simulink model "graduation_project_prototype_collect_4"  (R2023a)
settings: Solver=VariableStepAuto  StartTime=0.0  StopTime=2  MaxStep=5e-3  RelTol=1e-3
libraries: spsFourierLib x10, slpidlib x3, spsAsynchronousMachineSIUnitsLib x1, spsDCVoltageSourceLib x1, spsPWMGenerator2LevelLib x1, spsSVPWMGenerator2LevelLib x1, spsabctoAlphaBetaZeroLib x1, spsabctodq0Lib x1, spsdq0toAlphaBetaZeroLib x1, spsThreePhaseVIMeasurementLib x1, spsTwoLevelConverterLib x1, sps_lib x1
settings Model: SimulationMode=accelerator  Creator=ehabt  LastModifiedBy=mohammed
settings DataIOCC: SaveOutput=off  SignalLogging=off  DSMLogging=off  SaveTime=off  ReturnWorkspaceOutputs=off

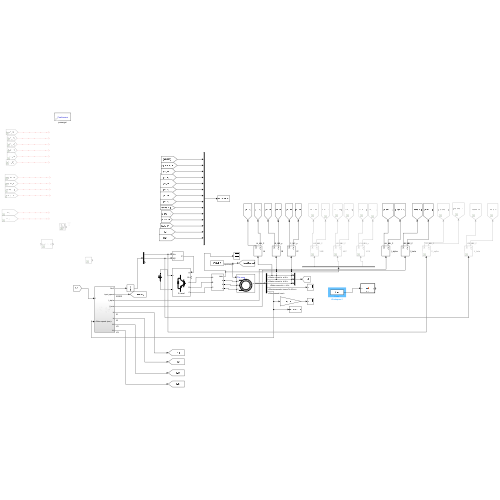
[thumbnail: Simulink's stored preview of the top-level diagram]
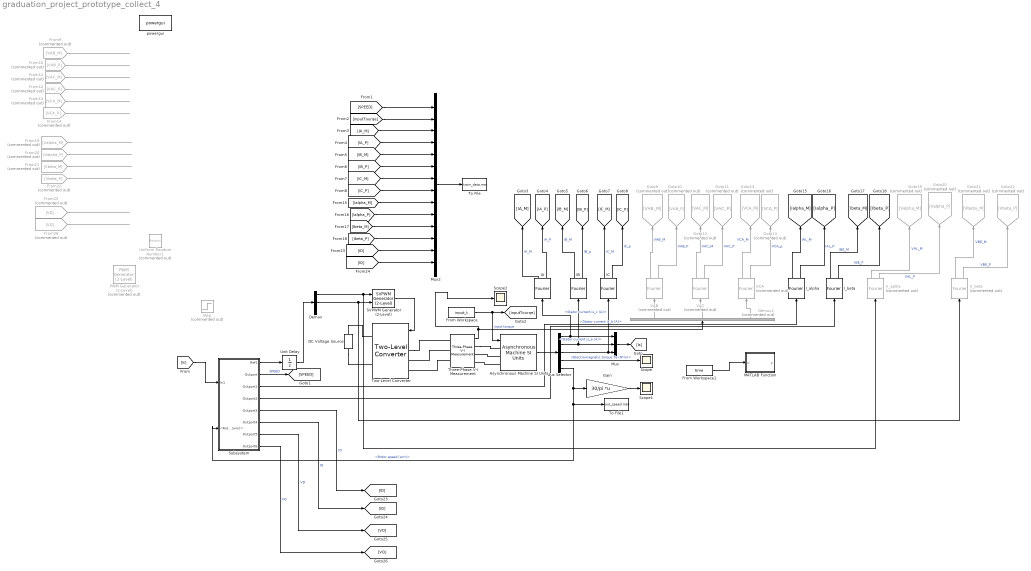
== system graduation_project_prototype_collect_4 ==
  Asynchronous Machine SI Units : spsAsynchronousMachineSIUnitsLib/Asynchronous Machine SI Units  RotorType=Squirrel-cage  PresetModel=No  MechanicalLoad=Torque Tm  ShowDetailedParameters=on  ReferenceFrame=Rotor  Units=SI  MeasurementBus=off  NominalParameters=[4000 400 50]  VoltageRatio=1  Stator=[1.405 0.005839]  Rotor=[1.395 0.005839]  Cage1=[0.4155 0.002066]  Cage2=[0.4168 0.0003495]  Lm=0.1722  Mechanical=[0.0131*3 0.002985 2]  PolePairs=2  InitialConditions=[1 0 0 0 0 0 0 0]  SimulateSaturation=off  Saturation=[14.03593122, 27.81365428, 53.79336849, 72.68890987, 97.98006896, 148.6815601, 215.7428561, 302.9841135, 428.7778367 ; 230, 322, 414, 460, 506, 552, 598, 644, 690]  LoadFlowParameters=1492000  TsPowergui=0  TsBlock=-1  IterativeModel=Trapezoidal non iterative  IterativeDiscreteModel=Trapezoidal non iterative  Pmec=1.492e+006
  Bus Selector : BusSelector  OutputSignals=Stator measurements.Stator current is_a (A),Stator measurements.Stator current is_b (A),Stator measurements.Stator current is_c (A),Mechanical.Electromagnetic torque Te (N*m),Mechanical.Rotor speed (wm)
  DC Voltage Source : spsDCVoltageSourceLib/DC Voltage Source  Amplitude=660  Measurements=None
  Demux : Demux  Outputs=3
  Demux1 : Demux  Commented=on  Outputs=3
  From Workspace : FromWorkspace  VariableName=input_t  SampleTime=2
  From Workspace1 : FromWorkspace  VariableName=time  SampleTime=1
  From10 : From  Commented=on  GotoTag=VAB_P
  From11 : From  Commented=on  GotoTag=VAC_M
  From12 : From  Commented=on  GotoTag=VAC_P
  From13 : From  Commented=on  GotoTag=VCA_M
  From14 : From  Commented=on  GotoTag=VCA_P
  From19 : From  Commented=on  GotoTag=Valpha_M
  From20 : From  Commented=on  GotoTag=Valpha_P
  From21 : From  Commented=on  GotoTag=Vbeta_M
  From22 : From  Commented=on  GotoTag=Vbeta_P
  From25 : From  Commented=on  GotoTag=VD
  From26 : From  Commented=on  GotoTag=VQ
  From9 : From  Commented=on  GotoTag=VAB_M
  Gain : Gain  Gain=30/pi  Multiplication=Matrix(K*u)
  Goto10 : Goto  Commented=on  GotoTag=VAB_P
  Goto11 : Goto  Commented=on  GotoTag=VAC_P
  Goto12 : Goto  Commented=on  GotoTag=VAC_M
  Goto13 : Goto  Commented=on  GotoTag=VCA_P
  Goto14 : Goto  Commented=on  GotoTag=VCA_M
  Goto19 : Goto  Commented=on  GotoTag=Valpha_M
  Goto20 : Goto  Commented=on  GotoTag=Valpha_P
  Goto21 : Goto  Commented=on  GotoTag=Vbeta_M
  Goto22 : Goto  Commented=on  GotoTag=Vbeta_P
  Goto9 : Goto  Commented=on  GotoTag=VAB_M
  IA : spsFourierLib/Fourier  Freq=50  n=1  InInit=[0, 0]  Ts=0
  IB : spsFourierLib/Fourier  Freq=50  n=1  InInit=[0, 0]  Ts=0
  IC : spsFourierLib/Fourier  Freq=50  n=1  InInit=[0, 0]  Ts=0
  I_alpha : spsFourierLib/Fourier  Freq=50  n=1  InInit=[0, 0]  Ts=0
  I_beta : spsFourierLib/Fourier  Freq=50  n=1  InInit=[0, 0]  Ts=0
  MATLAB Function : MATLAB Function  TreatAsAtomicUnit=on
  Mux : Mux  Inputs=3
  Mux2 : Mux  Inputs=14
  PWM Generator (2-Level) : spsPWMGenerator2LevelLib/PWM Generator (2-Level)  Commented=on  ModulatorType=Three-phase bridge (6 pulses)  ModulatorMode=Unsynchronized  Fc=5000  Pc=90  nF=27  MinMax="[ -1  1 ]"  SamplingTechnique=Natural  ModulatingSignals=off  m=0.8  Freq=60  Phase=0  Ts=0  ShowCarrierOutport=off
  SVPWM Generator (2-Level) : spsSVPWMGenerator2LevelLib/SVPWM Generator (2-Level)  InputType=alpha-beta components  SwitchingPattern=Pattern #1  Fc=15000  ParUref=[0.8 -30 50]  Ts=0
  Scope : Scope
  Scope1 : Scope
  Scope2 : Scope
  Step : Step  Commented=on  After=26  SampleTime=0
  Subsystem : Subsystem
  Three-Phase V-I Measurement : spsThreePhaseVIMeasurementLib/Three-Phase V-I Measurement  VoltageMeasurement=phase-to-phase  SetLabelV=off  LabelV=Vabc  Vpu=off  VpuLL=off  CurrentMeasurement=no  SetLabelI=off  LabelI=Iabc  Ipu=off  Pbase=100e6  Vbase=500e3  OutputType=Complex  PhasorSimulation=off  PSBequivalent=0
  To File : ToFile  Filename=train_data.mat  MatrixName=train_data  SaveFormat=Timeseries  SampleTime=1.99
  To File1 : ToFile  Filename=out_speed.mat  MatrixName=out_speed  SaveFormat=Timeseries  SampleTime=1.99
  Two-Level Converter : spsTwoLevelConverterLib/Two-Level Converter  ModelType=Switching devices  Ron=1e-3  Rs=1e6  Cs=inf  Vforward=[0,0]  Ron_Diode=1e-3  Rs_Diode=1e6  Cs_Diode=inf  Vf_Diode=1e-3  Rs_CurrentSource=inf  Ron_ACsource=1e-3
      settings: LibrarySourceBlock=sps_lib/Power Electronics/Two-Level Converter
  Uniform Random Number1 : UniformRandomNumber  Commented=on  Minimum=0  Maximum=26  Seed=1234  SampleTime=2
  Unit Delay : UnitDelay  SampleTime=-1  HasFrameUpgradeWarning=on
  VAB : spsFourierLib/Fourier  Commented=on  Freq=50  n=1  InInit=[0, 0]  Ts=0
  VAC : spsFourierLib/Fourier  Commented=on  Freq=50  n=1  InInit=[0, 0]  Ts=0
  VCA : spsFourierLib/Fourier  Commented=on  Freq=50  n=1  InInit=[0, 0]  Ts=0
  V_aplha : spsFourierLib/Fourier  Commented=on  Freq=50  n=1  InInit=[0, 0]  Ts=0
  V_beta : spsFourierLib/Fourier  Commented=on  Freq=50  n=1  InInit=[0, 0]  Ts=0
  powergui : sps_lib/powergui  Priority=1  SimulationMode=Continuous  SampleTime=50e-6  frequency=60  Iterations=50  frequencyindice=50  Pbase=100e6  ErrMax=1e-4  UnitsV=kV  UnitsW=MW  buscounter=0  FunctionMessages=off  echomessages=off  EnableUseOfTLC=off  CurrentSourceSwitches=off  DisableSnubberDevices=off  DisableRonSwitches=off  DisableVfSwitches=off  DisplayEquations=off  AutomaticDiscreteSolvers=off  SolverType=Tustin/Backward Euler (TBE)  Interpol=off  ExternalGateDelay=off  methode=off  Ts=100  x0status=blocks  SPID=on  SwTol=0  HookPort=off  NonlinearTolerance=1e-4  nMaxIteration=100  ContinueOnMaxIteration=off  RestoreLinks=warning  ResistiveCurrentMeasurement=off  Frange=[0:2:500]  Ylog=off  Xlog=on  ShowGrid=off  save=off  variable=ZData  structure=0  ZoomFFT=off  StartTime=0.0  cycles=1  DisplayStyle=1  fundamental=60  FreqAxis=off  MaxFrequency=1000  frequencyindicesteady=1  RmsSteady=1  display=off
  wires:
  Asynchronous Machine SI Units/1 -> Bus Selector/1
  Bus Selector/1 -> Mux/1, IA/1  "<Stator current is_a (A)>"
  Bus Selector/2 -> Mux/2, IB/1  "<Stator current is_b (A)>"
  Bus Selector/3 -> IC/1, Mux/3  "<Stator current is_c (A)>"
  Bus Selector/4 -> Scope/1  "<Electromagnetic torque Te (N*m)>"
  Mux/1 -> [Is]
  Bus Selector/5 -> To File1/1, Subsystem/2(<Rotor speed (wm)>), Gain/1  "<Rotor speed (wm)>"
  Gain/1 -> Scope1/1
  [Is] -> Subsystem/1(In1)
  Three-Phase V-I Measurement/1 -> Demux1/1, Scope2/1
  Subsystem/1(Ref1) -> Unit Delay/1
  Unit Delay/1 -> Demux/1
  Demux/1 -> V_aplha/1, SVPWM Generator (2-Level)/1
  Demux/2 -> V_beta/1, SVPWM Generator (2-Level)/2
  SVPWM Generator (2-Level)/1 -> Two-Level Converter/1
  From Workspace/1 -> Asynchronous Machine SI Units/1, [inputTourqe]  "input torque"
  Demux1/1 -> VAB/1
  Demux1/2 -> VAC/1
  Demux1/3 -> VCA/1
  Subsystem/3(Outport1) -> I_alpha/1
  Subsystem/4(Outport2) -> I_beta/1
  Subsystem/2(Outport) -> [SPEED]  "SPEED"
  [SPEED] -> Mux2/1
  [inputTourqe] -> Mux2/2
  IA/1 -> [IA_M]  "IA_M"
  IA/2 -> [IA_P]  "IA_P"
  IB/1 -> [IB_M]  "IB_M"
  IB/2 -> [IB_P]  "IB_p"
  IC/1 -> [IC_M]  "IC_M"
  IC/2 -> [IC_P]  "IC_p"
  VAB/1 -> Goto9/1  "VAB_M"
  VAB/2 -> Goto10/1  "VAB_P"
  VAC/1 -> Goto12/1  "VAC_M"
  VAC/2 -> Goto11/1  "VAC_P"
  VCA/1 -> Goto14/1  "VCA_M"
  VCA/2 -> Goto13/1  "VCA_p"
  I_alpha/1 -> [Ialpha_M]  "IAL_M"
  I_alpha/2 -> [Ialpha_P]  "IAL_P"
  I_beta/1 -> [Ibeta_M]  "IBE_M"
  I_beta/2 -> [Ibeta_P]  "IBE_P"
  V_aplha/1 -> Goto19/1  "VAL_M"
  V_aplha/2 -> Goto20/1  "VAL_P"
  V_beta/1 -> Goto21/1  "VBE_M"
  V_beta/2 -> Goto22/1  "VBE_P"
  Subsystem/5(Outport3) -> [ID]  "ID"
  Subsystem/6(Outport4) -> [IQ]  "IQ"
  Subsystem/7(Outport5) -> [VD]  "VD"
  Subsystem/8(Outport6) -> [VQ]  "VQ"
  [IA_M] -> Mux2/3
  [IA_P] -> Mux2/4
  [IB_M] -> Mux2/5
  [IB_P] -> Mux2/6
  [IC_M] -> Mux2/7
  [IC_P] -> Mux2/8
  From9/1 -> ?
  From10/1 -> ?
  From11/1 -> ?
  From12/1 -> ?
  From13/1 -> ?
  From14/1 -> ?
  [Ialpha_M] -> Mux2/9
  [Ialpha_P] -> Mux2/10
  [Ibeta_M] -> Mux2/11
  [Ibeta_P] -> Mux2/12
  From19/1 -> ?
  From20/1 -> ?
  From21/1 -> ?
  From22/1 -> ?
  [ID] -> Mux2/13
  [IQ] -> Mux2/14
  From25/1 -> ?
  From26/1 -> ?
  Mux2/1 -> To File/1
  From Workspace1/1 -> MATLAB Function/1(u)
  connections:
  Asynchronous Machine SI Units/LConn2 -- Three-Phase V-I Measurement/RConn2
  Asynchronous Machine SI Units/LConn3 -- Three-Phase V-I Measurement/RConn3
  DC Voltage Source/RConn1 -- Two-Level Converter/RConn1
  DC Voltage Source/LConn1 -- Two-Level Converter/RConn2
  Three-Phase V-I Measurement/LConn2 -- Two-Level Converter/LConn2
  Three-Phase V-I Measurement/LConn3 -- Two-Level Converter/LConn3
  Three-Phase V-I Measurement/RConn1 -- Asynchronous Machine SI Units/LConn1
  Two-Level Converter/LConn1 -- Three-Phase V-I Measurement/LConn1

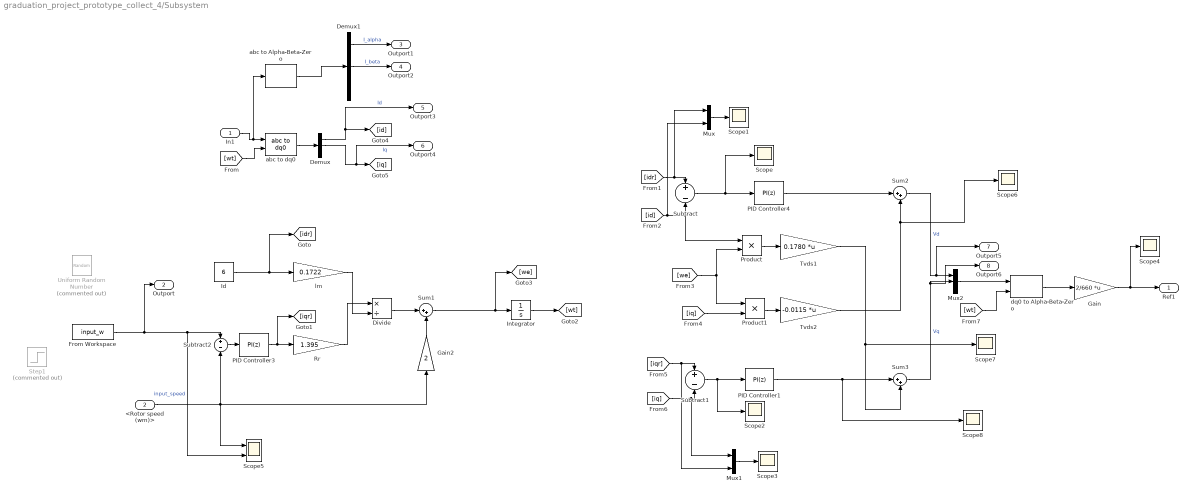
== system graduation_project_prototype_collect_4/Subsystem ==
  In1 : Inport
  <Rotor speed (wm)> : Inport  Port=2
  Demux : Demux  Outputs=3
  Demux1 : Demux  Outputs=3
  Divide : Product  Inputs=*/
  From Workspace : FromWorkspace  VariableName=input_w  SampleTime=2
  Gain : Gain  Gain=2/660  Multiplication=Matrix(K*u)
  Gain2 : Gain  Gain=2
  Id : Constant  Value=6
  Integrator : Integrator
  Mux : Mux  Inputs=2
  Mux1 : Mux  Inputs=2
  Mux2 : Mux  Inputs=3
  PID Controller1 : slpidlib/PID Controller  Controller=PI  Form=Parallel  TimeDomain=Discrete-time  UseExternalTs=off  SampleTime=100e-6  IntegratorMethod=Forward Euler  FilterMethod=Forward Euler  ControllerParametersSource=internal  P=6.66265142907135  I=1139.27458602713  UseKiTs=off  D=0  N=100  UseFilter=on  TunerSelectOption=Transfer Function Based (PID Tuner App)  InitialConditionSource=internal  InitialConditionForIntegrator=0  InitialConditionForFilter=0  DifferentiatorICPrevScaledInput=0  ExternalReset=none  TrackingMode=off  Kt=1  LimitOutput=on  SatLimitsSource=internal  UpperSaturationLimit=330  LowerSaturationLimit=-330  LinearizeAsGain=on  AntiWindupMode=clamping  Kb=1  LimitIntegrator=off  UpperIntegratorSaturationLimit=inf  LowerIntegratorSaturationLimit=-inf  POutMin=[]  POutMax=[]  IOutMin=[]  IOutMax=[]  DOutMin=[]  DOutMax=[]  NOutMin=[]  NOutMax=[]  SumOutMin=[]  SumOutMax=[]  SaturationOutMin=[]  SaturationOutMax=[]  PParamMin=[]  PParamMax=[]  IParamMin=[]  IParamMax=[]  DParamMin=[]  DParamMax=[]  NParamMin=[]  NParamMax=[]  KbParamMin=[]  KbParamMax=[]  KtParamMin=[]  KtParamMax=[]  KbOutMin=[]  KbOutMax=[]  KtOutMin=[]  KtOutMax=[]  IntegratorOutMin=[]  IntegratorOutMax=[]  FilterOutMin=[]  FilterOutMax=[]  SumI1OutMin=[]  SumI1OutMax=[]  SumI2OutMin=[]  SumI2OutMax=[]  SumI3OutMin=[]  SumI3OutMax=[]  SumI4OutMin=[]  SumI4OutMax=[]  SumDOutMin=[]  SumDOutMax=[]  DifferentiatorOutMin=[]  DifferentiatorOutMax=[]  FilterDiffOutCoefMin=[]  FilterDiffOutCoefMax=[]  ReciprocalOutMin=[]  ReciprocalOutMax=[]  SumDenOutMin=[]  SumDenOutMax=[]  SumNumOutMin=[]  SumNumOutMax=[]  DivideOutMin=[]  DivideOutMax=[]  UdiffTsProdOutMin=[]  UdiffTsProdOutMax=[]  NTsProdOutMin=[]  NTsProdOutMax=[]  UintegralTsProdOutMin=[]  UintegralTsProdOutMax=[]  UngainTsProdOutMin=[]  UngainTsProdOutMax=[]  ClampingZeroOutDataTypeStr=Inherit: Inherit via back propagation  ClampingZeroOutMin=[]  ClampingZeroOutMax=[]  FilterDenConstantOutDataTypeStr=Inherit: Inherit via back propagation  FilterDenConstantOutMin=[]  FilterDenConstantOutMax=[]  PCopyOutDataTypeStr=Inherit: Inherit via back propagation  PCopyOutMin=[]  PCopyOutMax=[]  NCopyOutDataTypeStr=Inherit: Inherit via back propagation  NCopyOutMin=[]  NCopyOutMax=[]  IntegratorContinuousStateAttributes=''  IntegratorStateMustResolveToSignalObject=off  IntegratorRTWStateStorageClass=Auto  FilterContinuousStateAttributes=''  FilterStateMustResolveToSignalObject=off  FilterRTWStateStorageClass=Auto  ParallelPVariant=InternalParameters  IdealPVariant=Disabled  IVariant=InternalParameters  DVariant=Disabled  IntegratorVariant=Discrete  SatVariant=Enabled  AWVariant=DiscClampingParallel  PCopyVariant=Disabled  TRVariant=Disabled  FdbkBlocksVariant=Forward  IdealPFdbkVariant=Disabled  SatFdbkVariant=Disabled  DerivativeFilterVariant=Disabled  NVariant=Disabled  NCopyVariant=Disabled_SignalSpec  FilterICVariant=Disabled  IntegratorICVariant=InternalICs  ExternalResetVariant=Disabled  TRSumVariant=Passthrough  SumFdbkVariant=Disabled  SumVariant=Sum_PI  TsampFilterVariant=InternalTs  TsampNgainVariant=Passthrough  TsampIntegralVariant=Disabled_SignalSpec  ExternalSaturationOutDataTypeStr=Inherit: Same as second input
  PID Controller3 : slpidlib/PID Controller  Controller=PI  Form=Parallel  TimeDomain=Discrete-time  UseExternalTs=off  SampleTime=100e-6  IntegratorMethod=Forward Euler  FilterMethod=Forward Euler  ControllerParametersSource=internal  P=1.27476437850265  I=15.6272018921627  UseKiTs=off  D=0  N=100  UseFilter=on  TunerSelectOption=Transfer Function Based (PID Tuner App)  InitialConditionSource=internal  InitialConditionForIntegrator=0  InitialConditionForFilter=0  DifferentiatorICPrevScaledInput=0  ExternalReset=none  TrackingMode=off  Kt=1  LimitOutput=on  SatLimitsSource=internal  UpperSaturationLimit=18  LowerSaturationLimit=-18  LinearizeAsGain=on  AntiWindupMode=clamping  Kb=1  LimitIntegrator=off  UpperIntegratorSaturationLimit=inf  LowerIntegratorSaturationLimit=-inf  POutMin=[]  POutMax=[]  IOutMin=[]  IOutMax=[]  DOutMin=[]  DOutMax=[]  NOutMin=[]  NOutMax=[]  SumOutMin=[]  SumOutMax=[]  SaturationOutMin=[]  SaturationOutMax=[]  PParamMin=[]  PParamMax=[]  IParamMin=[]  IParamMax=[]  DParamMin=[]  DParamMax=[]  NParamMin=[]  NParamMax=[]  KbParamMin=[]  KbParamMax=[]  KtParamMin=[]  KtParamMax=[]  KbOutMin=[]  KbOutMax=[]  KtOutMin=[]  KtOutMax=[]  IntegratorOutMin=[]  IntegratorOutMax=[]  FilterOutMin=[]  FilterOutMax=[]  SumI1OutMin=[]  SumI1OutMax=[]  SumI2OutMin=[]  SumI2OutMax=[]  SumI3OutMin=[]  SumI3OutMax=[]  SumI4OutMin=[]  SumI4OutMax=[]  SumDOutMin=[]  SumDOutMax=[]  DifferentiatorOutMin=[]  DifferentiatorOutMax=[]  FilterDiffOutCoefMin=[]  FilterDiffOutCoefMax=[]  ReciprocalOutMin=[]  ReciprocalOutMax=[]  SumDenOutMin=[]  SumDenOutMax=[]  SumNumOutMin=[]  SumNumOutMax=[]  DivideOutMin=[]  DivideOutMax=[]  UdiffTsProdOutMin=[]  UdiffTsProdOutMax=[]  NTsProdOutMin=[]  NTsProdOutMax=[]  UintegralTsProdOutMin=[]  UintegralTsProdOutMax=[]  UngainTsProdOutMin=[]  UngainTsProdOutMax=[]  ClampingZeroOutDataTypeStr=Inherit: Inherit via back propagation  ClampingZeroOutMin=[]  ClampingZeroOutMax=[]  FilterDenConstantOutDataTypeStr=Inherit: Inherit via back propagation  FilterDenConstantOutMin=[]  FilterDenConstantOutMax=[]  PCopyOutDataTypeStr=Inherit: Inherit via back propagation  PCopyOutMin=[]  PCopyOutMax=[]  NCopyOutDataTypeStr=Inherit: Inherit via back propagation  NCopyOutMin=[]  NCopyOutMax=[]  IntegratorContinuousStateAttributes=''  IntegratorStateMustResolveToSignalObject=off  IntegratorRTWStateStorageClass=Auto  FilterContinuousStateAttributes=''  FilterStateMustResolveToSignalObject=off  FilterRTWStateStorageClass=Auto  ParallelPVariant=InternalParameters  IdealPVariant=Disabled  IVariant=InternalParameters  DVariant=Disabled  IntegratorVariant=Discrete  SatVariant=Enabled  AWVariant=DiscClampingParallel  PCopyVariant=Disabled  TRVariant=Disabled  FdbkBlocksVariant=Forward  IdealPFdbkVariant=Disabled  SatFdbkVariant=Disabled  DerivativeFilterVariant=Disabled  NVariant=Disabled  NCopyVariant=Disabled_SignalSpec  FilterICVariant=Disabled  IntegratorICVariant=InternalICs  ExternalResetVariant=Disabled  TRSumVariant=Passthrough  SumFdbkVariant=Disabled  SumVariant=Sum_PI  TsampFilterVariant=InternalTs  TsampNgainVariant=Passthrough  TsampIntegralVariant=Disabled_SignalSpec  ExternalSaturationOutDataTypeStr=Inherit: Same as second input
  PID Controller4 : slpidlib/PID Controller  Controller=PI  Form=Parallel  TimeDomain=Discrete-time  UseExternalTs=off  SampleTime=100e-6  IntegratorMethod=Forward Euler  FilterMethod=Forward Euler  ControllerParametersSource=internal  P=12.2885137139008  I=162.749993865987  UseKiTs=off  D=0  N=100  UseFilter=on  TunerSelectOption=Transfer Function Based (PID Tuner App)  InitialConditionSource=internal  InitialConditionForIntegrator=0  InitialConditionForFilter=0  DifferentiatorICPrevScaledInput=0  ExternalReset=none  TrackingMode=off  Kt=1  LimitOutput=on  SatLimitsSource=internal  UpperSaturationLimit=330  LowerSaturationLimit=-330  LinearizeAsGain=on  AntiWindupMode=clamping  Kb=1  LimitIntegrator=off  UpperIntegratorSaturationLimit=inf  LowerIntegratorSaturationLimit=-inf  POutMin=[]  POutMax=[]  IOutMin=[]  IOutMax=[]  DOutMin=[]  DOutMax=[]  NOutMin=[]  NOutMax=[]  SumOutMin=[]  SumOutMax=[]  SaturationOutMin=[]  SaturationOutMax=[]  PParamMin=[]  PParamMax=[]  IParamMin=[]  IParamMax=[]  DParamMin=[]  DParamMax=[]  NParamMin=[]  NParamMax=[]  KbParamMin=[]  KbParamMax=[]  KtParamMin=[]  KtParamMax=[]  KbOutMin=[]  KbOutMax=[]  KtOutMin=[]  KtOutMax=[]  IntegratorOutMin=[]  IntegratorOutMax=[]  FilterOutMin=[]  FilterOutMax=[]  SumI1OutMin=[]  SumI1OutMax=[]  SumI2OutMin=[]  SumI2OutMax=[]  SumI3OutMin=[]  SumI3OutMax=[]  SumI4OutMin=[]  SumI4OutMax=[]  SumDOutMin=[]  SumDOutMax=[]  DifferentiatorOutMin=[]  DifferentiatorOutMax=[]  FilterDiffOutCoefMin=[]  FilterDiffOutCoefMax=[]  ReciprocalOutMin=[]  ReciprocalOutMax=[]  SumDenOutMin=[]  SumDenOutMax=[]  SumNumOutMin=[]  SumNumOutMax=[]  DivideOutMin=[]  DivideOutMax=[]  UdiffTsProdOutMin=[]  UdiffTsProdOutMax=[]  NTsProdOutMin=[]  NTsProdOutMax=[]  UintegralTsProdOutMin=[]  UintegralTsProdOutMax=[]  UngainTsProdOutMin=[]  UngainTsProdOutMax=[]  ClampingZeroOutDataTypeStr=Inherit: Inherit via back propagation  ClampingZeroOutMin=[]  ClampingZeroOutMax=[]  FilterDenConstantOutDataTypeStr=Inherit: Inherit via back propagation  FilterDenConstantOutMin=[]  FilterDenConstantOutMax=[]  PCopyOutDataTypeStr=Inherit: Inherit via back propagation  PCopyOutMin=[]  PCopyOutMax=[]  NCopyOutDataTypeStr=Inherit: Inherit via back propagation  NCopyOutMin=[]  NCopyOutMax=[]  IntegratorContinuousStateAttributes=''  IntegratorStateMustResolveToSignalObject=off  IntegratorRTWStateStorageClass=Auto  FilterContinuousStateAttributes=''  FilterStateMustResolveToSignalObject=off  FilterRTWStateStorageClass=Auto  ParallelPVariant=InternalParameters  IdealPVariant=Disabled  IVariant=InternalParameters  DVariant=Disabled  IntegratorVariant=Discrete  SatVariant=Enabled  AWVariant=DiscClampingParallel  PCopyVariant=Disabled  TRVariant=Disabled  FdbkBlocksVariant=Forward  IdealPFdbkVariant=Disabled  SatFdbkVariant=Disabled  DerivativeFilterVariant=Disabled  NVariant=Disabled  NCopyVariant=Disabled_SignalSpec  FilterICVariant=Disabled  IntegratorICVariant=InternalICs  ExternalResetVariant=Disabled  TRSumVariant=Passthrough  SumFdbkVariant=Disabled  SumVariant=Sum_PI  TsampFilterVariant=InternalTs  TsampNgainVariant=Passthrough  TsampIntegralVariant=Disabled_SignalSpec  ExternalSaturationOutDataTypeStr=Inherit: Same as second input
  Product : Product
  Product1 : Product
  Rr : Gain  Gain=1.395
  Scope{,1..4,6..8} (8 alike) : Scope
  Scope5 : Scope  NumInputPorts=2
  Step1 : Step  Commented=on  Time=0.2  After=1250*pi/30  SampleTime=0
  Subtract : Sum  Inputs=+-
  Subtract1 : Sum  Inputs=+-
  Subtract2 : Sum  Inputs=+-
  Sum1 : Sum  Inputs=|++
  Sum2 : Sum  Inputs=|++
  Sum3 : Sum  Inputs=|++
  Tvds1 : Gain  Gain=0.1780  Multiplication=Matrix(K*u)
  Tvds2 : Gain  Gain=-0.0115  Multiplication=Matrix(K*u)
  Uniform Random Number : UniformRandomNumber  Commented=on  Minimum=0  Maximum=1500*pi/30  Seed=1234  SampleTime=2
  abc to Alpha-Beta-Zero : spsabctoAlphaBetaZeroLib/abc to Alpha-Beta-Zero
  abc to dq0 : spsabctodq0Lib/abc to dq0  Alignment=90 degrees behind phase A axis
  dq0 to Alpha-Beta-Zero : spsdq0toAlphaBetaZeroLib/dq0 to Alpha-Beta-Zero  Alignment=90 degrees behind phase A axis
  lm : Gain  Gain=0.1722
  Ref1 : Outport
  Outport : Outport  Port=2
  Outport1 : Outport  Port=3
  Outport2 : Outport  Port=4
  Outport3 : Outport  Port=5
  Outport4 : Outport  Port=6
  Outport5 : Outport  Port=7
  Outport6 : Outport  Port=8
  wires:
  <Rotor speed (wm)>/1 -> Subtract2/2, Scope5/1, Gain2/1
  Rr/1 -> Divide/1
  Id/1 -> [idr], lm/1
  lm/1 -> Divide/2
  Divide/1 -> Sum1/1
  Sum1/1 -> [we], Integrator/1
  Integrator/1 -> [wt]
  Subtract2/1 -> PID Controller3/1
  PID Controller3/1 -> [iqr], Rr/1
  In1/1 -> abc to Alpha-Beta-Zero/1, abc to dq0/1
  [wt] -> abc to dq0/2
  abc to dq0/1 -> Demux/1
  Demux/1 -> Outport3/1, [id]  "Id"
  [idr] -> Mux/1, Subtract/1
  Subtract/1 -> PID Controller4/1, Scope/1
  [id] -> Subtract/2, Product/1, Mux/2
  Mux/1 -> Scope1/1
  [we] -> Product1/1, Product/2
  [iq] -> Product1/2
  [iqr] -> Mux1/2, Subtract1/1
  [iq] -> Mux1/1, Subtract1/2
  Subtract1/1 -> PID Controller1/1, Scope2/1
  Mux1/1 -> Scope3/1
  Product/1 -> Tvds1/1
  Product1/1 -> Tvds2/1
  PID Controller4/1 -> Sum2/1
  Tvds2/1 -> Scope6/1, Sum2/2
  Tvds1/1 -> Scope7/1, Sum3/2
  PID Controller1/1 -> Scope8/1, Sum3/1
  Sum2/1 -> Outport5/1, Mux2/1  "Vd"
  Sum3/1 -> Outport6/1, Mux2/2  "Vq"
  [wt] -> dq0 to Alpha-Beta-Zero/2
  dq0 to Alpha-Beta-Zero/1 -> Gain/1
  Gain/1 -> Scope4/1, Ref1/1
  Demux/2 -> Outport4/1, [iq]  "Iq"
  Mux2/1 -> dq0 to Alpha-Beta-Zero/1
  From Workspace/1 -> Outport/1, Scope5/2, Subtract2/1  "input_speed"
  abc to Alpha-Beta-Zero/1 -> Demux1/1
  Demux1/1 -> Outport1/1  "I_alpha"
  Demux1/2 -> Outport2/1  "I_beta"
  Gain2/1 -> Sum1/2

== matlab function graduation_project_prototype_collect_4/MATLAB Function ==
  data: u input; y output
function y = fcn(u)

disp(u);
y = 0;
